simulink model "help"  (R2020a)
settings: Solver=FixedStepAuto  StartTime=0.0  StopTime=10.0  FixedStep=1e-3  RelTol=1e-3  EnableMultiTasking=on
libraries: frdmk64flib x9
settings Model: ExtModeTrigDuration=5  Creator=qasim  LastModifiedBy=qasim
settings OptimizationCC: EnhancedBackFolding=on  PassReuseOutputArgsAs=Individual arguments  ZeroExternalMemoryAtStartup=off  ZeroInternalMemoryAtStartup=off  MaxStackSize=64  OptimizeBlockOrder=speed  DifferentSizesBufferReuse=on  OptimizationCustomize=off  EfficientTunableParamExpr=on
settings DebuggingCC: ParameterTunabilityLossMsg=error
settings HardwareCC: ProdBitPerPointer=32  ProdBitPerSizeT=32  ProdBitPerPtrDiffT=32  ProdLargestAtomicInteger=Long  ProdLargestAtomicFloat=Double  ProdWordSize=32  ProdHWDeviceType=ARM Compatible->ARM Cortex
settings SFSimCC: MATLABDynamicMemAlloc=off
settings RTWCC: SystemTargetFile=ert.tlc  HardwareBoard=NXP FRDM-K64F  TemplateMakefile=ert_default_tmf  Toolchain=GNU Tools for ARM Embedded Processors
settings CodeAppCC: ForceParamTrailComments=on  IgnoreCustomStorageClasses=off  OperatorAnnotations=on  SimulinkDataObjDesc=on  SFDataObjDesc=on  InsertBlockDesc=on

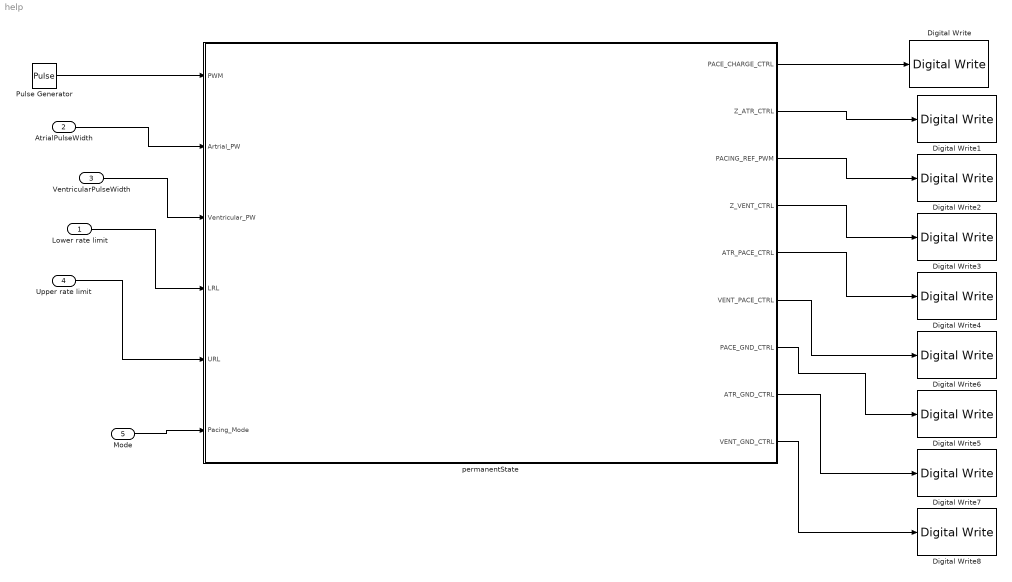
== system help ==
  Lower rate limit : Inport
  AtrialPulseWidth : Inport  Port=2
  VentricularPulseWidth : Inport  Port=3
  Upper rate limit : Inport  Port=4
  Mode : Inport  Port=5
  Digital Write{,1..8} (9 alike) : frdmk64flib/Digital Write  Whichpin=RED_LED
  Pulse Generator : DiscretePulseGenerator  PulseType=Time based  Period=1/2000  PulseWidth=5
  permanentState : Stateflow chart  TreatAsAtomicUnit=on
  wires:
  Pulse Generator/1 -> permanentState/1(PWM)
  Lower rate limit/1 -> permanentState/4(LRL)
  VentricularPulseWidth/1 -> permanentState/3(Ventricular_PW)
  Upper rate limit/1 -> permanentState/5(URL)
  Mode/1 -> permanentState/6(Pacing_Mode)
  AtrialPulseWidth/1 -> permanentState/2(Artrial_PW)
  permanentState/1(PACE_CHARGE_CTRL) -> Digital Write/1
  permanentState/2(Z_ATR_CTRL) -> Digital Write1/1
  permanentState/3(PACING_REF_PWM) -> Digital Write2/1
  permanentState/4(Z_VENT_CTRL) -> Digital Write3/1
  permanentState/5(ATR_PACE_CTRL) -> Digital Write4/1
  permanentState/6(VENT_PACE_CTRL) -> Digital Write6/1
  permanentState/7(PACE_GND_CTRL) -> Digital Write5/1
  permanentState/8(ATR_GND_CTRL) -> Digital Write7/1
  permanentState/9(VENT_GND_CTRL) -> Digital Write8/1

== stateflow chart help/permanentState ==
  state AXX_charging
    entry:
    PACE_CHARGE_CTRL = 0
    Z_ATR_CTRL = 0;
    ATR_PACE_CTRL= 0;
    ATR_GND_CTRL= 1;
    PACE_GND_CTRL= 1;
    PACING_REF_PWM= 0;
  state AXX_pacing
    entry:
    PACE_CHARGE_CTRL = 0
    Z_ATR_CTRL = 0;
    ATR_PACE_CTRL= 1;
    ATR_GND_CTRL= 0;
    PACE_GND_CTRL= 1;
    PACING_REF_PWM= 0;
  state INIT
    entry:
    PACE_CHARGE_CTRL = 1;
    Z_ATR_CTRL= 0;
    PACING_REF_PWM= PWM;
    Z_VENT_CTRL = 0;
    ATR_PACE_CTRL = 0;
    VENT_PACE_CTRL = 0;
    PACE_GND_CTRL = 0;
    ATR_GND_CTRL = 0;
    VENT_GND_CTRL = 0;
  state VXX_pacing
    entry:
    PACE_CHARGE_CTRL = 0
    Z_ATR_CTRL = 0;
    Vent_PACE_CTRL= 1;
    Vent_GND_CTRL= 0;
    PACE_GND_CTRL= 1;
    PACING_REF_PWM= 0;
  state VXX_charging
    entry:
    PACE_CHARGE_CTRL = 0
    Z_ATR_CTRL = 0;
    Vent_PACE_CTRL= 0;
    Vent_GND_CTRL= 1;
    PACE_GND_CTRL= 1;
    PACING_REF_PWM= 0;
  AXX_charging -> AXX_pacing : [after(Artrial_PW,msec)]
  AXX_pacing -> AXX_charging : [after(Artrial_PW,msec)]
  (default) -> INIT
  VXX_charging -> VXX_pacing : [after(Ventricular_PW,msec)]
  VXX_pacing -> VXX_charging : [after(Ventricular_PW,msec)]
  data: PWM input; Artrial_PW input; Ventricular_PW input; LRL input; URL input; Pacing_Mode input; PACE_CHARGE_CTRL output; Z_ATR_CTRL output; PACING_REF_PWM output; Z_VENT_CTRL output; ATR_PACE_CTRL output; VENT_PACE_CTRL output; PACE_GND_CTRL output; ATR_GND_CTRL output; VENT_GND_CTRL output
